simulink model "PENDULO"  (R2024b)
settings: Solver=VariableStepAuto  StartTime=0.0  StopTime=40  RelTol=1e-3
libraries: simulink x2
settings Model: Creator=RREYM  LastModifiedBy=RREYM

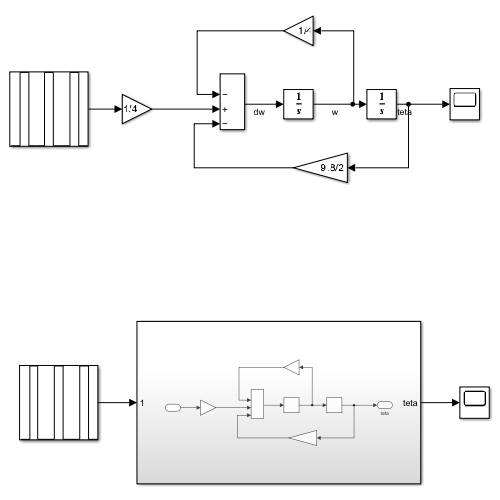
[thumbnail: Simulink's stored preview of the top-level diagram]
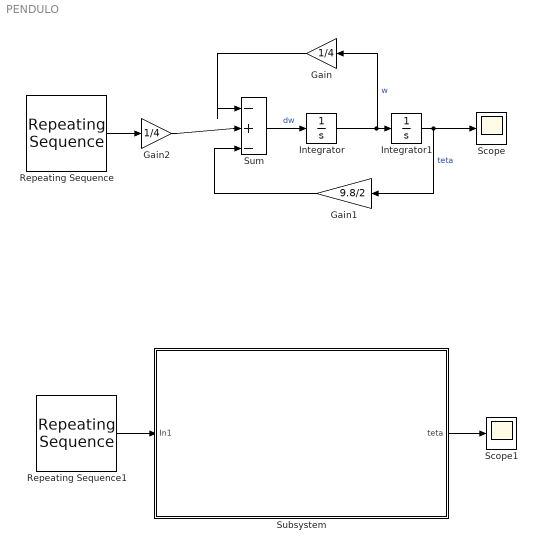
== system PENDULO ==
  Gain : Gain  Gain=1/4
  Gain1 : Gain  Gain=9.8/2
  Gain2 : Gain  Gain=1/4
  Integrator : Integrator
  Integrator1 : Integrator
  Repeating Sequence : simulink/Sources/Repeating Sequence  rep_seq_t=[0 1 1.001 2 2.001 3]  rep_seq_y=[0 0 1 1 0 0]
  Repeating Sequence1 : simulink/Sources/Repeating Sequence  rep_seq_t=[0 1 1.001 2 2.001 3]  rep_seq_y=[0 0 1 1 0 0]
  Scope : Scope
  Scope1 : Scope
  Subsystem : Subsystem
  Sum : Sum  Inputs=|-+-
  wires:
  Integrator/1 -> Gain/1, Integrator1/1  "w"
  Integrator1/1 -> Scope/1, Gain1/1  "teta"
  Sum/1 -> Integrator/1  "dw"
  Gain1/1 -> Sum/3
  Gain/1 -> Sum/1
  Gain2/1 -> Sum/2
  Repeating Sequence/1 -> Gain2/1
  Repeating Sequence1/1 -> Subsystem/1(In1)
  Subsystem/1(teta) -> Scope1/1

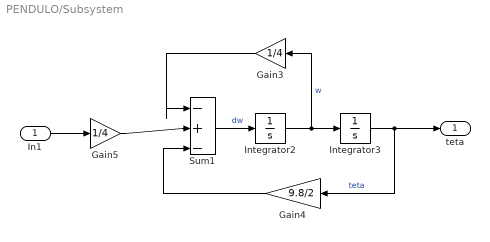
== system PENDULO/Subsystem ==
  In1 : Inport
  Gain3 : Gain  Gain=1/4
  Gain4 : Gain  Gain=9.8/2
  Gain5 : Gain  Gain=1/4
  Integrator2 : Integrator
  Integrator3 : Integrator
  Sum1 : Sum  Inputs=|-+-
  teta : Outport
  wires:
  Integrator3/1 -> teta/1, Gain4/1  "teta"
  Gain4/1 -> Sum1/3
  Sum1/1 -> Integrator2/1  "dw"
  In1/1 -> Gain5/1
  Integrator2/1 -> Gain3/1, Integrator3/1  "w"
  Gain3/1 -> Sum1/1
  Gain5/1 -> Sum1/2
